simulink model "first_order_accel"  (R2023b)
settings: Solver=VariableStepAuto  StartTime=0.0  StopTime=30.0  RelTol=1e-3
libraries: simulink x1
settings Model: Creator=Maxwe  LastModifiedBy=Maxwe
settings HardwareCC: ProdHWDeviceType=AMD->x86-64 (Windows64)

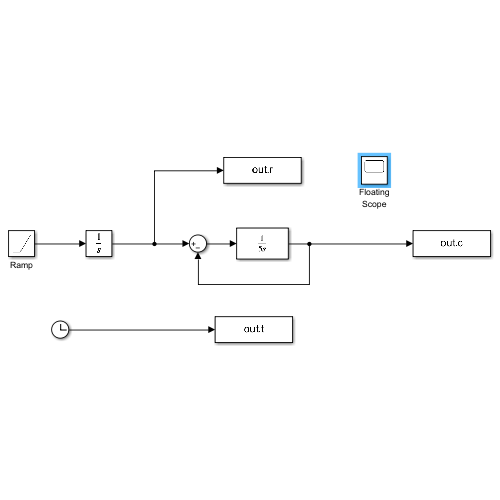
[thumbnail: Simulink's stored preview of the top-level diagram]
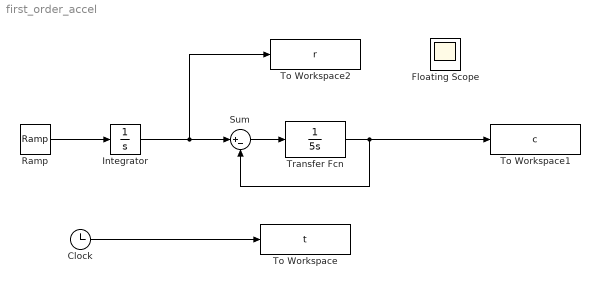
== system first_order_accel ==
  Clock : Clock
  Floating Scope : Scope
      settings: Floating=on
  Integrator : Integrator
  Ramp : simulink/Sources/Ramp  slope=1  start=0  InitialOutput=0
  Sum : Sum  Inputs=|+-
  To Workspace : ToWorkspace  VariableName=t  SampleTime=-1
      settings: Save2DSignal=2-D array (concatenate along first dimension)
  To Workspace1 : ToWorkspace  VariableName=c  SampleTime=-1
      settings: Save2DSignal=2-D array (concatenate along first dimension)
  To Workspace2 : ToWorkspace  VariableName=r  SampleTime=-1
      settings: Save2DSignal=2-D array (concatenate along first dimension)
  Transfer Fcn : TransferFcn  Denominator=[5 0]
  wires:
  Sum/1 -> Transfer Fcn/1
  Ramp/1 -> Integrator/1
  Transfer Fcn/1 -> To Workspace1/1, Sum/2
  Clock/1 -> To Workspace/1
  Integrator/1 -> Sum/1, To Workspace2/1
